simulink model "P1"  (R2019a)
settings: Solver=VariableStepAuto  StartTime=0.0  StopTime=10.0  RelTol=1e-3
settings Model: Creator=ADMIN  LastModifiedBy=ADMIN

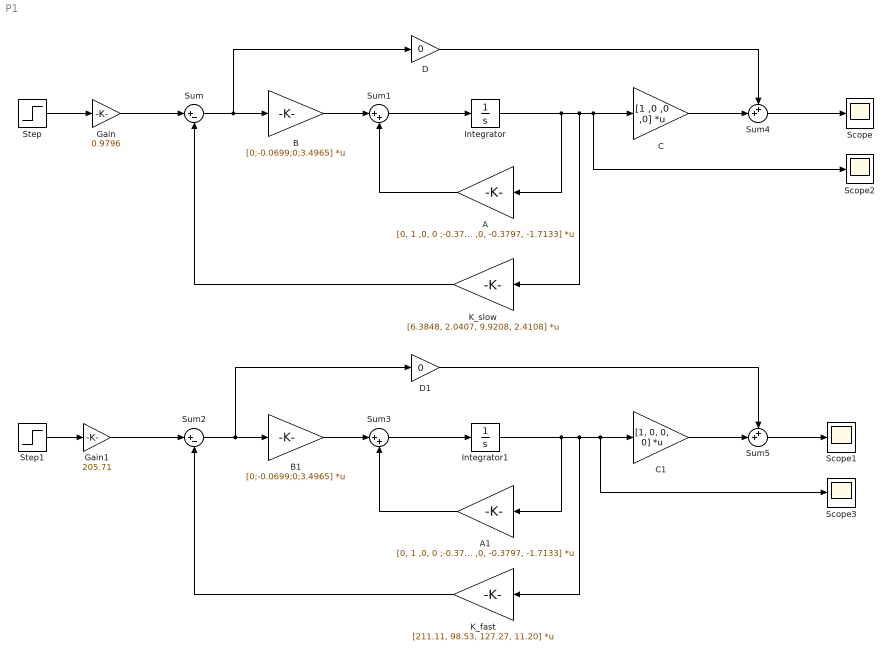
== system P1 ==
  A : Gain  Gain=[0, 1 ,0, 0 ;-0.378 ,0 ,7.0147 ,0.0343;0, 0, 0, 1; 18.9001 ,0, -0.3797, -1.7133]  Multiplication=Matrix(K*u) (u vector)
  A1 : Gain  Gain=[0, 1 ,0, 0 ;-0.378 ,0 ,7.0147 ,0.0343;0, 0, 0, 1; 18.9001 ,0, -0.3797, -1.7133]  Multiplication=Matrix(K*u) (u vector)
  B : Gain  Gain=[0;-0.0699;0;3.4965]  Multiplication=Matrix(K*u) (u vector)
  B1 : Gain  Gain=[0;-0.0699;0;3.4965]  Multiplication=Matrix(K*u) (u vector)
  C : Gain  Gain=[1 ,0 ,0 ,0]  Multiplication=Matrix(K*u) (u vector)
  C1 : Gain  Gain=[1, 0, 0, 0]  Multiplication=Matrix(K*u) (u vector)
  D : Gain  Gain=0
  D1 : Gain  Gain=0
  Gain : Gain  Gain=0.9796
  Gain1 : Gain  Gain=205.71
  Integrator : Integrator
  Integrator1 : Integrator
  K_fast : Gain  Gain=[211.11, 98.53, 127.27, 11.20]  Multiplication=Matrix(K*u) (u vector)
  K_slow : Gain  Gain=[6.3848, 2.0407, 9.9208, 2.4108]  Multiplication=Matrix(K*u) (u vector)
  Scope{,1..3} (4 alike) : Scope
  Step : Step  Time=0  After=0.1  SampleTime=0
  Step1 : Step  Time=0  After=0.1  SampleTime=0
  Sum : Sum  Inputs=|+-
  Sum1 : Sum  Inputs=|++
  Sum2 : Sum  Inputs=|+-
  Sum3 : Sum  Inputs=|++
  Sum4 : Sum  Inputs=++|
  Sum5 : Sum  Inputs=++|
  wires:
  Integrator/1 -> A/1, Scope2/1, C/1, K_slow/1
  K_slow/1 -> Sum/2
  B/1 -> Sum1/1
  Sum1/1 -> Integrator/1
  Sum/1 -> B/1, D/1
  A/1 -> Sum1/2
  K_fast/1 -> Sum2/2
  A1/1 -> Sum3/2
  Sum3/1 -> Integrator1/1
  B1/1 -> Sum3/1
  C/1 -> Sum4/2
  D/1 -> Sum4/1
  Sum4/1 -> Scope/1
  Sum5/1 -> Scope1/1
  D1/1 -> Sum5/1
  C1/1 -> Sum5/2
  Sum2/1 -> B1/1, D1/1
  Integrator1/1 -> A1/1, Scope3/1, C1/1, K_fast/1
  Step/1 -> Gain/1
  Gain/1 -> Sum/1
  Gain1/1 -> Sum2/1
  Step1/1 -> Gain1/1
